simulink model "assignment5"  (R2017b)
settings: Solver=VariableStepAuto  StartTime=0.0  StopTime=10.0  RelTol=1e-3
libraries: hdlsllib x17
settings Model: Creator=Raymond  LastModifiedBy=Ray

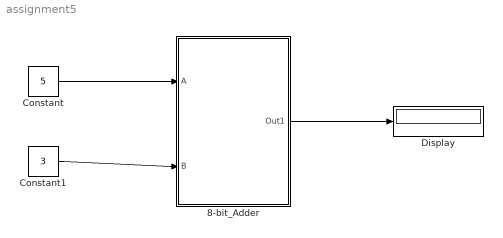
== system assignment5 ==
  8-bit_Adder : Subsystem
  Constant : Constant  Value=5  OutDataTypeStr=int8  SampleTime=-1
  Constant1 : Constant  Value=3  OutDataTypeStr=int8  SampleTime=-1
  Display : Display
  wires:
  Constant/1 -> 8-bit_Adder/1(A)
  Constant1/1 -> 8-bit_Adder/2(B)
  8-bit_Adder/1(Out1) -> Display/1

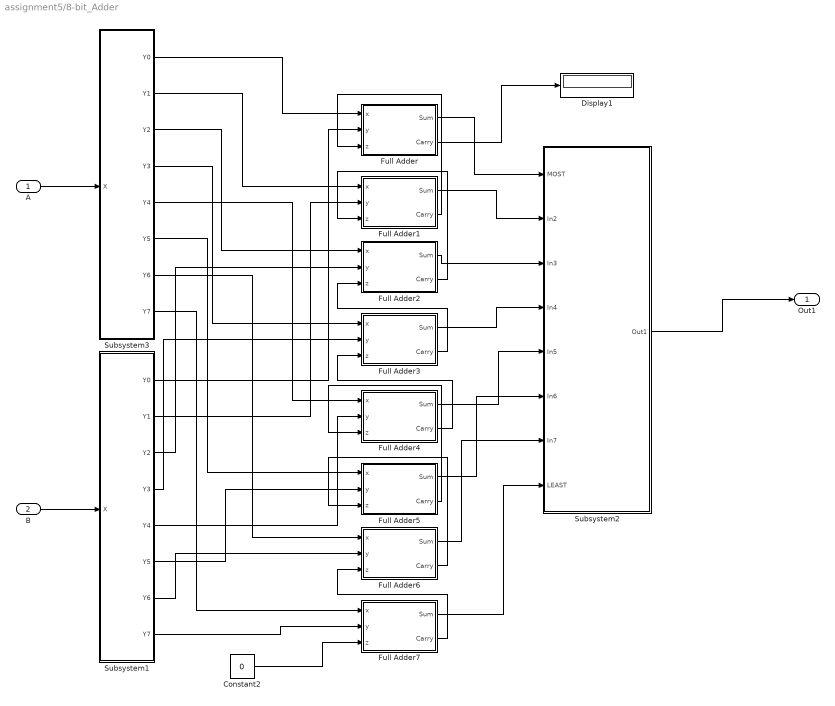
== system assignment5/8-bit_Adder ==
  A : Inport
  B : Inport  Port=2
  Constant2 : Constant  Value=0  OutDataTypeStr=int8  SampleTime=-1
  Display1 : Display
  Full Adder : Subsystem
  Full Adder1 : Subsystem
  Full Adder2 : Subsystem
  Full Adder3 : Subsystem
  Full Adder4 : Subsystem
  Full Adder5 : Subsystem
  Full Adder6 : Subsystem
  Full Adder7 : Subsystem
  Subsystem1 : Subsystem
  Subsystem2 : Subsystem
  Subsystem3 : Subsystem
  Out1 : Outport
  wires:
  A/1 -> Subsystem3/1(X)
  B/1 -> Subsystem1/1(X)
  Subsystem3/1(Y0) -> Full Adder/1(x)
  Subsystem3/2(Y1) -> Full Adder1/1(x)
  Subsystem3/3(Y2) -> Full Adder2/1(x)
  Subsystem3/4(Y3) -> Full Adder3/1(x)
  Subsystem3/5(Y4) -> Full Adder4/1(x)
  Subsystem3/6(Y5) -> Full Adder5/1(x)
  Subsystem3/7(Y6) -> Full Adder6/1(x)
  Subsystem3/8(Y7) -> Full Adder7/1(x)
  Subsystem1/1(Y0) -> Full Adder/2(y)
  Subsystem1/2(Y1) -> Full Adder1/2(y)
  Subsystem1/3(Y2) -> Full Adder2/2(y)
  Subsystem1/4(Y3) -> Full Adder3/2(y)
  Subsystem1/5(Y4) -> Full Adder4/2(y)
  Subsystem1/6(Y5) -> Full Adder5/2(y)
  Subsystem1/7(Y6) -> Full Adder6/2(y)
  Subsystem1/8(Y7) -> Full Adder7/2(y)
  Constant2/1 -> Full Adder7/3(z)
  Full Adder7/2(Carry) -> Full Adder6/3(z)
  Full Adder6/2(Carry) -> Full Adder5/3(z)
  Full Adder5/2(Carry) -> Full Adder4/3(z)
  Full Adder4/2(Carry) -> Full Adder3/3(z)
  Full Adder3/2(Carry) -> Full Adder2/3(z)
  Full Adder2/2(Carry) -> Full Adder1/3(z)
  Full Adder1/2(Carry) -> Full Adder/3(z)
  Subsystem2/1(Out1) -> Out1/1
  Full Adder/2(Carry) -> Display1/1
  Full Adder2/1(Sum) -> Subsystem2/3(In3)
  Full Adder3/1(Sum) -> Subsystem2/4(In4)
  Full Adder1/1(Sum) -> Subsystem2/2(In2)
  Full Adder4/1(Sum) -> Subsystem2/5(In5)
  Full Adder/1(Sum) -> Subsystem2/1(MOST)
  Full Adder5/1(Sum) -> Subsystem2/6(In6)
  Full Adder6/1(Sum) -> Subsystem2/7(In7)
  Full Adder7/1(Sum) -> Subsystem2/8(LEAST)

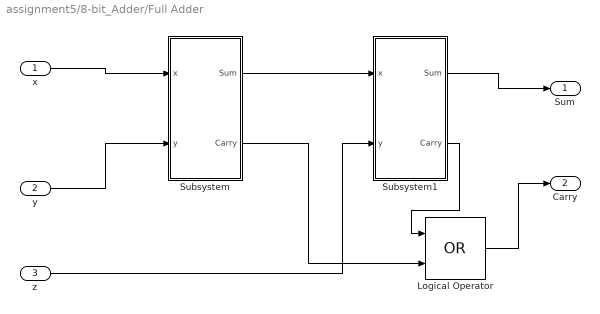
== system assignment5/8-bit_Adder/Full Adder ==
  x : Inport
  y : Inport  Port=2
  z : Inport  Port=3
  Logical Operator : Logic  Operator=OR  IconShape=distinctive  AllPortsSameDT=off  OutDataTypeStr=boolean
  Subsystem : Subsystem
  Subsystem1 : Subsystem
  Sum : Outport
  Carry : Outport  Port=2
  wires:
  z/1 -> Subsystem1/2(y)
  Subsystem/2(Carry) -> Logical Operator/2
  Subsystem1/1(Sum) -> Sum/1
  x/1 -> Subsystem/1(x)
  y/1 -> Subsystem/2(y)
  Subsystem/1(Sum) -> Subsystem1/1(x)
  Subsystem1/2(Carry) -> Logical Operator/1
  Logical Operator/1 -> Carry/1

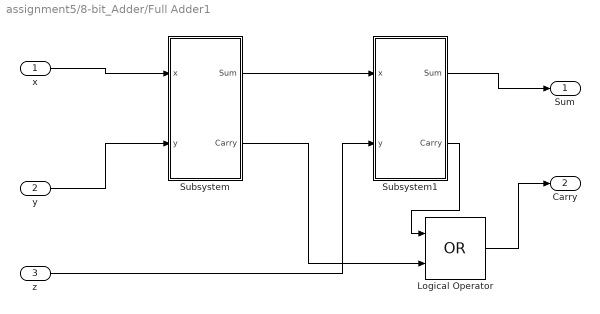
== system assignment5/8-bit_Adder/Full Adder1 ==
  x : Inport
  y : Inport  Port=2
  z : Inport  Port=3
  Logical Operator : Logic  Operator=OR  IconShape=distinctive  AllPortsSameDT=off  OutDataTypeStr=boolean
  Subsystem : Subsystem
  Subsystem1 : Subsystem
  Sum : Outport
  Carry : Outport  Port=2
  wires:
  z/1 -> Subsystem1/2(y)
  Subsystem/2(Carry) -> Logical Operator/2
  Subsystem1/1(Sum) -> Sum/1
  x/1 -> Subsystem/1(x)
  y/1 -> Subsystem/2(y)
  Subsystem/1(Sum) -> Subsystem1/1(x)
  Subsystem1/2(Carry) -> Logical Operator/1
  Logical Operator/1 -> Carry/1

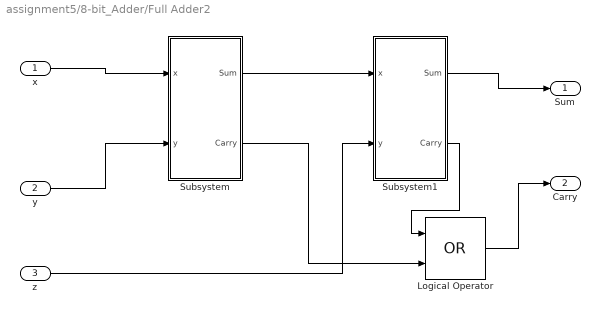
== system assignment5/8-bit_Adder/Full Adder2 ==
  x : Inport
  y : Inport  Port=2
  z : Inport  Port=3
  Logical Operator : Logic  Operator=OR  IconShape=distinctive  AllPortsSameDT=off  OutDataTypeStr=boolean
  Subsystem : Subsystem
  Subsystem1 : Subsystem
  Sum : Outport
  Carry : Outport  Port=2
  wires:
  z/1 -> Subsystem1/2(y)
  Subsystem/2(Carry) -> Logical Operator/2
  Subsystem1/1(Sum) -> Sum/1
  x/1 -> Subsystem/1(x)
  y/1 -> Subsystem/2(y)
  Subsystem/1(Sum) -> Subsystem1/1(x)
  Subsystem1/2(Carry) -> Logical Operator/1
  Logical Operator/1 -> Carry/1

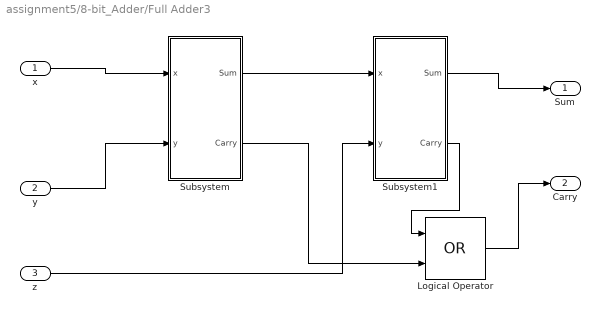
== system assignment5/8-bit_Adder/Full Adder3 ==
  x : Inport
  y : Inport  Port=2
  z : Inport  Port=3
  Logical Operator : Logic  Operator=OR  IconShape=distinctive  AllPortsSameDT=off  OutDataTypeStr=boolean
  Subsystem : Subsystem
  Subsystem1 : Subsystem
  Sum : Outport
  Carry : Outport  Port=2
  wires:
  Logical Operator/1 -> Carry/1
  Subsystem1/2(Carry) -> Logical Operator/1
  Subsystem/1(Sum) -> Subsystem1/1(x)
  y/1 -> Subsystem/2(y)
  x/1 -> Subsystem/1(x)
  Subsystem1/1(Sum) -> Sum/1
  Subsystem/2(Carry) -> Logical Operator/2
  z/1 -> Subsystem1/2(y)

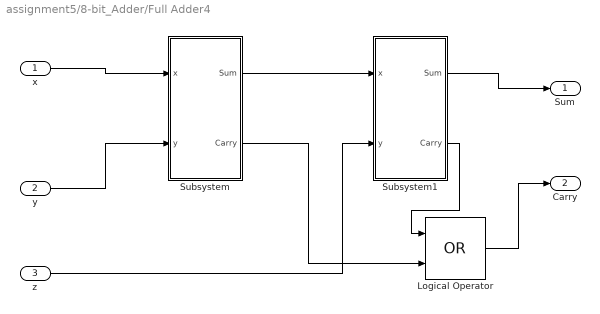
== system assignment5/8-bit_Adder/Full Adder4 ==
  x : Inport
  y : Inport  Port=2
  z : Inport  Port=3
  Logical Operator : Logic  Operator=OR  IconShape=distinctive  AllPortsSameDT=off  OutDataTypeStr=boolean
  Subsystem : Subsystem
  Subsystem1 : Subsystem
  Sum : Outport
  Carry : Outport  Port=2
  wires:
  z/1 -> Subsystem1/2(y)
  Subsystem/2(Carry) -> Logical Operator/2
  Subsystem1/1(Sum) -> Sum/1
  x/1 -> Subsystem/1(x)
  y/1 -> Subsystem/2(y)
  Subsystem/1(Sum) -> Subsystem1/1(x)
  Subsystem1/2(Carry) -> Logical Operator/1
  Logical Operator/1 -> Carry/1

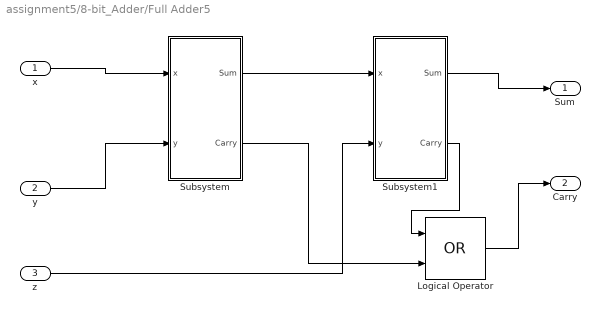
== system assignment5/8-bit_Adder/Full Adder5 ==
  x : Inport
  y : Inport  Port=2
  z : Inport  Port=3
  Logical Operator : Logic  Operator=OR  IconShape=distinctive  AllPortsSameDT=off  OutDataTypeStr=boolean
  Subsystem : Subsystem
  Subsystem1 : Subsystem
  Sum : Outport
  Carry : Outport  Port=2
  wires:
  z/1 -> Subsystem1/2(y)
  Subsystem/2(Carry) -> Logical Operator/2
  Subsystem1/1(Sum) -> Sum/1
  x/1 -> Subsystem/1(x)
  y/1 -> Subsystem/2(y)
  Subsystem/1(Sum) -> Subsystem1/1(x)
  Subsystem1/2(Carry) -> Logical Operator/1
  Logical Operator/1 -> Carry/1

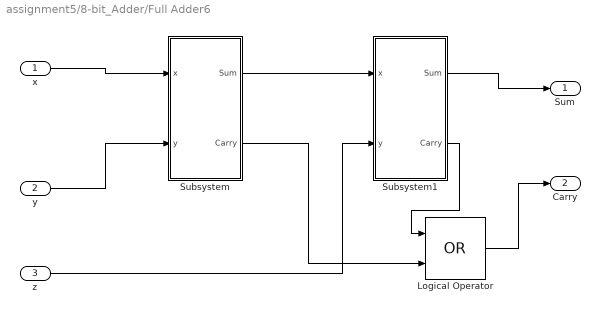
== system assignment5/8-bit_Adder/Full Adder6 ==
  x : Inport
  y : Inport  Port=2
  z : Inport  Port=3
  Logical Operator : Logic  Operator=OR  IconShape=distinctive  AllPortsSameDT=off  OutDataTypeStr=boolean
  Subsystem : Subsystem
  Subsystem1 : Subsystem
  Sum : Outport
  Carry : Outport  Port=2
  wires:
  z/1 -> Subsystem1/2(y)
  Subsystem/2(Carry) -> Logical Operator/2
  Subsystem1/1(Sum) -> Sum/1
  x/1 -> Subsystem/1(x)
  y/1 -> Subsystem/2(y)
  Subsystem/1(Sum) -> Subsystem1/1(x)
  Subsystem1/2(Carry) -> Logical Operator/1
  Logical Operator/1 -> Carry/1

== system assignment5/8-bit_Adder/Full Adder7 ==
  x : Inport
  y : Inport  Port=2
  z : Inport  Port=3
  Logical Operator : Logic  Operator=OR  IconShape=distinctive  AllPortsSameDT=off  OutDataTypeStr=boolean
  Subsystem : Subsystem
  Subsystem1 : Subsystem
  Sum : Outport
  Carry : Outport  Port=2
  wires:
  Logical Operator/1 -> Carry/1
  Subsystem1/2(Carry) -> Logical Operator/1
  Subsystem/1(Sum) -> Subsystem1/1(x)
  y/1 -> Subsystem/2(y)
  x/1 -> Subsystem/1(x)
  Subsystem1/1(Sum) -> Sum/1
  Subsystem/2(Carry) -> Logical Operator/2
  z/1 -> Subsystem1/2(y)

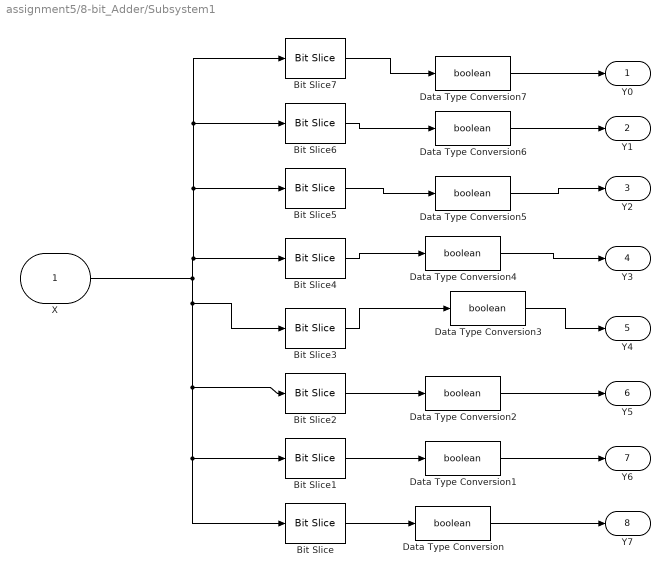
== system assignment5/8-bit_Adder/Subsystem1 ==
  X : Inport  OutDataTypeStr=int8  SampleTime=1
  Bit Slice : hdlsllib/Logic and Bit Operations/Bit Slice  lidx=0  ridx=0
  Bit Slice1 : hdlsllib/Logic and Bit Operations/Bit Slice  lidx=1  ridx=1
  Bit Slice2 : hdlsllib/Logic and Bit Operations/Bit Slice  lidx=2  ridx=2
  Bit Slice3 : hdlsllib/Logic and Bit Operations/Bit Slice  lidx=3  ridx=3
  Bit Slice4 : hdlsllib/Logic and Bit Operations/Bit Slice  lidx=4  ridx=4
  Bit Slice5 : hdlsllib/Logic and Bit Operations/Bit Slice  lidx=5  ridx=5
  Bit Slice6 : hdlsllib/Logic and Bit Operations/Bit Slice  lidx=6  ridx=6
  Bit Slice7 : hdlsllib/Logic and Bit Operations/Bit Slice  lidx=7  ridx=7
  Data Type Conversion{,1..7} (8 alike) : DataTypeConversion  OutDataTypeStr=boolean
  Y0 : Outport
  Y1 : Outport  Port=2
  Y2 : Outport  Port=3
  Y3 : Outport  Port=4
  Y4 : Outport  Port=5
  Y5 : Outport  Port=6
  Y6 : Outport  Port=7
  Y7 : Outport  Port=8
  wires:
  Data Type Conversion/1 -> Y7/1
  Data Type Conversion1/1 -> Y6/1
  Data Type Conversion6/1 -> Y1/1
  Bit Slice5/1 -> Data Type Conversion5/1
  Data Type Conversion5/1 -> Y2/1
  Data Type Conversion7/1 -> Y0/1
  X/1 -> Bit Slice/1, Bit Slice1/1, Bit Slice2/1, Bit Slice3/1, Bit Slice4/1, Bit Slice5/1, Bit Slice7/1, Bit Slice6/1
  Data Type Conversion3/1 -> Y4/1
  Data Type Conversion4/1 -> Y3/1
  Bit Slice2/1 -> Data Type Conversion2/1
  Bit Slice1/1 -> Data Type Conversion1/1
  Bit Slice/1 -> Data Type Conversion/1
  Data Type Conversion2/1 -> Y5/1
  Bit Slice7/1 -> Data Type Conversion7/1
  Bit Slice6/1 -> Data Type Conversion6/1
  Bit Slice4/1 -> Data Type Conversion4/1
  Bit Slice3/1 -> Data Type Conversion3/1

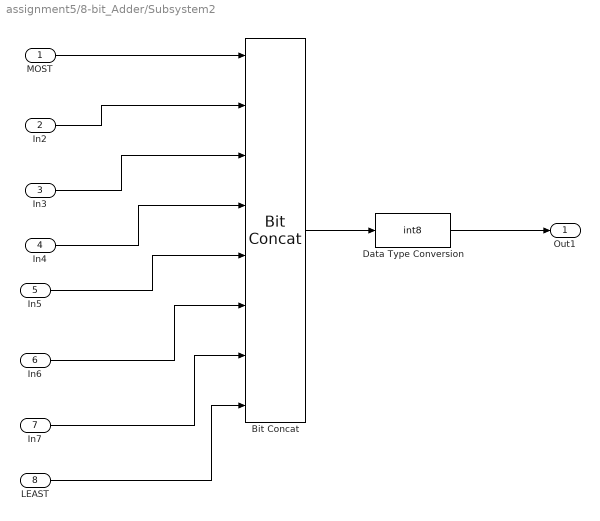
== system assignment5/8-bit_Adder/Subsystem2 ==
  MOST : Inport
  In2 : Inport  Port=2
  In3 : Inport  Port=3
  In4 : Inport  Port=4
  In5 : Inport  Port=5
  In6 : Inport  Port=6
  In7 : Inport  Port=7
  LEAST : Inport  Port=8
  Bit Concat : hdlsllib/Logic and Bit Operations/Bit Concat  numInputs=8
      settings: SourceProductName=HDL Coder  SourceProductBaseCode=HD
  Data Type Conversion : DataTypeConversion  OutDataTypeStr=int8
  Out1 : Outport
  wires:
  Bit Concat/1 -> Data Type Conversion/1
  Data Type Conversion/1 -> Out1/1
  In5/1 -> Bit Concat/5
  In6/1 -> Bit Concat/6
  MOST/1 -> Bit Concat/1
  In7/1 -> Bit Concat/7
  In3/1 -> Bit Concat/3
  In4/1 -> Bit Concat/4
  LEAST/1 -> Bit Concat/8
  In2/1 -> Bit Concat/2

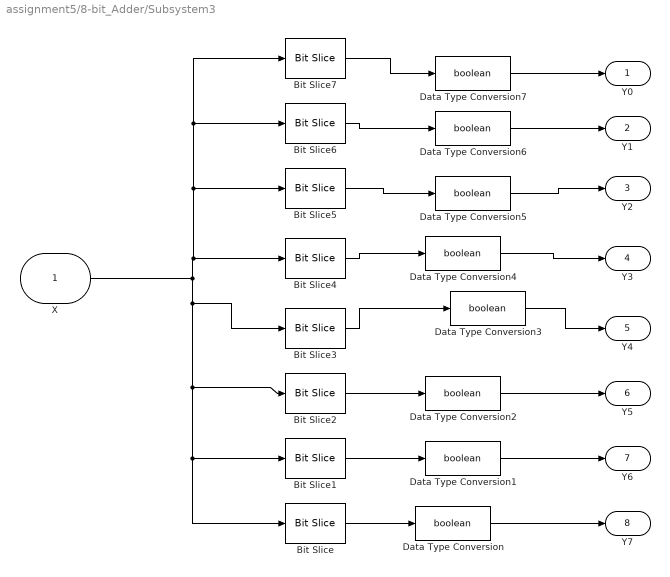
== system assignment5/8-bit_Adder/Subsystem3 ==
  X : Inport  OutDataTypeStr=int8  SampleTime=1
  Bit Slice : hdlsllib/Logic and Bit Operations/Bit Slice  lidx=0  ridx=0
  Bit Slice1 : hdlsllib/Logic and Bit Operations/Bit Slice  lidx=1  ridx=1
  Bit Slice2 : hdlsllib/Logic and Bit Operations/Bit Slice  lidx=2  ridx=2
  Bit Slice3 : hdlsllib/Logic and Bit Operations/Bit Slice  lidx=3  ridx=3
  Bit Slice4 : hdlsllib/Logic and Bit Operations/Bit Slice  lidx=4  ridx=4
  Bit Slice5 : hdlsllib/Logic and Bit Operations/Bit Slice  lidx=5  ridx=5
  Bit Slice6 : hdlsllib/Logic and Bit Operations/Bit Slice  lidx=6  ridx=6
  Bit Slice7 : hdlsllib/Logic and Bit Operations/Bit Slice  lidx=7  ridx=7
  Data Type Conversion{,1..7} (8 alike) : DataTypeConversion  OutDataTypeStr=boolean
  Y0 : Outport
  Y1 : Outport  Port=2
  Y2 : Outport  Port=3
  Y3 : Outport  Port=4
  Y4 : Outport  Port=5
  Y5 : Outport  Port=6
  Y6 : Outport  Port=7
  Y7 : Outport  Port=8
  wires:
  Data Type Conversion/1 -> Y7/1
  Data Type Conversion1/1 -> Y6/1
  Data Type Conversion6/1 -> Y1/1
  Bit Slice5/1 -> Data Type Conversion5/1
  Data Type Conversion5/1 -> Y2/1
  Data Type Conversion7/1 -> Y0/1
  X/1 -> Bit Slice/1, Bit Slice1/1, Bit Slice2/1, Bit Slice3/1, Bit Slice4/1, Bit Slice5/1, Bit Slice7/1, Bit Slice6/1
  Data Type Conversion3/1 -> Y4/1
  Data Type Conversion4/1 -> Y3/1
  Bit Slice2/1 -> Data Type Conversion2/1
  Bit Slice1/1 -> Data Type Conversion1/1
  Bit Slice/1 -> Data Type Conversion/1
  Data Type Conversion2/1 -> Y5/1
  Bit Slice7/1 -> Data Type Conversion7/1
  Bit Slice6/1 -> Data Type Conversion6/1
  Bit Slice4/1 -> Data Type Conversion4/1
  Bit Slice3/1 -> Data Type Conversion3/1

== system assignment5/8-bit_Adder/Full Adder/Subsystem ==
  x : Inport
  y : Inport  Port=2
  Logical Operator : Logic  IconShape=distinctive  AllPortsSameDT=off  OutDataTypeStr=boolean
  Logical Operator1 : Logic  Operator=XOR  IconShape=distinctive  AllPortsSameDT=off  OutDataTypeStr=boolean
  Sum : Outport
  Carry : Outport  Port=2
  wires:
  x/1 -> Logical Operator/1, Logical Operator1/1
  y/1 -> Logical Operator1/2, Logical Operator/2
  Logical Operator/1 -> Carry/1
  Logical Operator1/1 -> Sum/1

== system assignment5/8-bit_Adder/Full Adder/Subsystem1 ==
  x : Inport
  y : Inport  Port=2
  Logical Operator : Logic  IconShape=distinctive  AllPortsSameDT=off  OutDataTypeStr=boolean
  Logical Operator1 : Logic  Operator=XOR  IconShape=distinctive  AllPortsSameDT=off  OutDataTypeStr=boolean
  Sum : Outport
  Carry : Outport  Port=2
  wires:
  x/1 -> Logical Operator/1, Logical Operator1/1
  y/1 -> Logical Operator1/2, Logical Operator/2
  Logical Operator/1 -> Carry/1
  Logical Operator1/1 -> Sum/1

== system assignment5/8-bit_Adder/Full Adder1/Subsystem ==
  x : Inport
  y : Inport  Port=2
  Logical Operator : Logic  IconShape=distinctive  AllPortsSameDT=off  OutDataTypeStr=boolean
  Logical Operator1 : Logic  Operator=XOR  IconShape=distinctive  AllPortsSameDT=off  OutDataTypeStr=boolean
  Sum : Outport
  Carry : Outport  Port=2
  wires:
  x/1 -> Logical Operator/1, Logical Operator1/1
  y/1 -> Logical Operator1/2, Logical Operator/2
  Logical Operator/1 -> Carry/1
  Logical Operator1/1 -> Sum/1

== system assignment5/8-bit_Adder/Full Adder1/Subsystem1 ==
  x : Inport
  y : Inport  Port=2
  Logical Operator : Logic  IconShape=distinctive  AllPortsSameDT=off  OutDataTypeStr=boolean
  Logical Operator1 : Logic  Operator=XOR  IconShape=distinctive  AllPortsSameDT=off  OutDataTypeStr=boolean
  Sum : Outport
  Carry : Outport  Port=2
  wires:
  x/1 -> Logical Operator/1, Logical Operator1/1
  y/1 -> Logical Operator1/2, Logical Operator/2
  Logical Operator/1 -> Carry/1
  Logical Operator1/1 -> Sum/1

== system assignment5/8-bit_Adder/Full Adder2/Subsystem ==
  x : Inport
  y : Inport  Port=2
  Logical Operator : Logic  IconShape=distinctive  AllPortsSameDT=off  OutDataTypeStr=boolean
  Logical Operator1 : Logic  Operator=XOR  IconShape=distinctive  AllPortsSameDT=off  OutDataTypeStr=boolean
  Sum : Outport
  Carry : Outport  Port=2
  wires:
  x/1 -> Logical Operator/1, Logical Operator1/1
  y/1 -> Logical Operator1/2, Logical Operator/2
  Logical Operator/1 -> Carry/1
  Logical Operator1/1 -> Sum/1

== system assignment5/8-bit_Adder/Full Adder2/Subsystem1 ==
  x : Inport
  y : Inport  Port=2
  Logical Operator : Logic  IconShape=distinctive  AllPortsSameDT=off  OutDataTypeStr=boolean
  Logical Operator1 : Logic  Operator=XOR  IconShape=distinctive  AllPortsSameDT=off  OutDataTypeStr=boolean
  Sum : Outport
  Carry : Outport  Port=2
  wires:
  x/1 -> Logical Operator/1, Logical Operator1/1
  y/1 -> Logical Operator1/2, Logical Operator/2
  Logical Operator/1 -> Carry/1
  Logical Operator1/1 -> Sum/1

== system assignment5/8-bit_Adder/Full Adder3/Subsystem ==
  x : Inport
  y : Inport  Port=2
  Logical Operator : Logic  IconShape=distinctive  AllPortsSameDT=off  OutDataTypeStr=boolean
  Logical Operator1 : Logic  Operator=XOR  IconShape=distinctive  AllPortsSameDT=off  OutDataTypeStr=boolean
  Sum : Outport
  Carry : Outport  Port=2
  wires:
  Logical Operator1/1 -> Sum/1
  Logical Operator/1 -> Carry/1
  y/1 -> Logical Operator/2, Logical Operator1/2
  x/1 -> Logical Operator1/1, Logical Operator/1

== system assignment5/8-bit_Adder/Full Adder3/Subsystem1 ==
  x : Inport
  y : Inport  Port=2
  Logical Operator : Logic  IconShape=distinctive  AllPortsSameDT=off  OutDataTypeStr=boolean
  Logical Operator1 : Logic  Operator=XOR  IconShape=distinctive  AllPortsSameDT=off  OutDataTypeStr=boolean
  Sum : Outport
  Carry : Outport  Port=2
  wires:
  Logical Operator1/1 -> Sum/1
  Logical Operator/1 -> Carry/1
  y/1 -> Logical Operator/2, Logical Operator1/2
  x/1 -> Logical Operator1/1, Logical Operator/1

== system assignment5/8-bit_Adder/Full Adder4/Subsystem ==
  x : Inport
  y : Inport  Port=2
  Logical Operator : Logic  IconShape=distinctive  AllPortsSameDT=off  OutDataTypeStr=boolean
  Logical Operator1 : Logic  Operator=XOR  IconShape=distinctive  AllPortsSameDT=off  OutDataTypeStr=boolean
  Sum : Outport
  Carry : Outport  Port=2
  wires:
  x/1 -> Logical Operator/1, Logical Operator1/1
  y/1 -> Logical Operator1/2, Logical Operator/2
  Logical Operator/1 -> Carry/1
  Logical Operator1/1 -> Sum/1

== system assignment5/8-bit_Adder/Full Adder4/Subsystem1 ==
  x : Inport
  y : Inport  Port=2
  Logical Operator : Logic  IconShape=distinctive  AllPortsSameDT=off  OutDataTypeStr=boolean
  Logical Operator1 : Logic  Operator=XOR  IconShape=distinctive  AllPortsSameDT=off  OutDataTypeStr=boolean
  Sum : Outport
  Carry : Outport  Port=2
  wires:
  x/1 -> Logical Operator/1, Logical Operator1/1
  y/1 -> Logical Operator1/2, Logical Operator/2
  Logical Operator/1 -> Carry/1
  Logical Operator1/1 -> Sum/1

== system assignment5/8-bit_Adder/Full Adder5/Subsystem ==
  x : Inport
  y : Inport  Port=2
  Logical Operator : Logic  IconShape=distinctive  AllPortsSameDT=off  OutDataTypeStr=boolean
  Logical Operator1 : Logic  Operator=XOR  IconShape=distinctive  AllPortsSameDT=off  OutDataTypeStr=boolean
  Sum : Outport
  Carry : Outport  Port=2
  wires:
  x/1 -> Logical Operator/1, Logical Operator1/1
  y/1 -> Logical Operator1/2, Logical Operator/2
  Logical Operator/1 -> Carry/1
  Logical Operator1/1 -> Sum/1

== system assignment5/8-bit_Adder/Full Adder5/Subsystem1 ==
  x : Inport
  y : Inport  Port=2
  Logical Operator : Logic  IconShape=distinctive  AllPortsSameDT=off  OutDataTypeStr=boolean
  Logical Operator1 : Logic  Operator=XOR  IconShape=distinctive  AllPortsSameDT=off  OutDataTypeStr=boolean
  Sum : Outport
  Carry : Outport  Port=2
  wires:
  x/1 -> Logical Operator/1, Logical Operator1/1
  y/1 -> Logical Operator1/2, Logical Operator/2
  Logical Operator/1 -> Carry/1
  Logical Operator1/1 -> Sum/1

== system assignment5/8-bit_Adder/Full Adder6/Subsystem ==
  x : Inport
  y : Inport  Port=2
  Logical Operator : Logic  IconShape=distinctive  AllPortsSameDT=off  OutDataTypeStr=boolean
  Logical Operator1 : Logic  Operator=XOR  IconShape=distinctive  AllPortsSameDT=off  OutDataTypeStr=boolean
  Sum : Outport
  Carry : Outport  Port=2
  wires:
  x/1 -> Logical Operator/1, Logical Operator1/1
  y/1 -> Logical Operator1/2, Logical Operator/2
  Logical Operator/1 -> Carry/1
  Logical Operator1/1 -> Sum/1

== system assignment5/8-bit_Adder/Full Adder6/Subsystem1 ==
  x : Inport
  y : Inport  Port=2
  Logical Operator : Logic  IconShape=distinctive  AllPortsSameDT=off  OutDataTypeStr=boolean
  Logical Operator1 : Logic  Operator=XOR  IconShape=distinctive  AllPortsSameDT=off  OutDataTypeStr=boolean
  Sum : Outport
  Carry : Outport  Port=2
  wires:
  x/1 -> Logical Operator/1, Logical Operator1/1
  y/1 -> Logical Operator1/2, Logical Operator/2
  Logical Operator/1 -> Carry/1
  Logical Operator1/1 -> Sum/1

== system assignment5/8-bit_Adder/Full Adder7/Subsystem ==
  x : Inport
  y : Inport  Port=2
  Logical Operator : Logic  IconShape=distinctive  AllPortsSameDT=off  OutDataTypeStr=boolean
  Logical Operator1 : Logic  Operator=XOR  IconShape=distinctive  AllPortsSameDT=off  OutDataTypeStr=boolean
  Sum : Outport
  Carry : Outport  Port=2
  wires:
  Logical Operator1/1 -> Sum/1
  Logical Operator/1 -> Carry/1
  y/1 -> Logical Operator/2, Logical Operator1/2
  x/1 -> Logical Operator1/1, Logical Operator/1

== system assignment5/8-bit_Adder/Full Adder7/Subsystem1 ==
  x : Inport
  y : Inport  Port=2
  Logical Operator : Logic  IconShape=distinctive  AllPortsSameDT=off  OutDataTypeStr=boolean
  Logical Operator1 : Logic  Operator=XOR  IconShape=distinctive  AllPortsSameDT=off  OutDataTypeStr=boolean
  Sum : Outport
  Carry : Outport  Port=2
  wires:
  Logical Operator1/1 -> Sum/1
  Logical Operator/1 -> Carry/1
  y/1 -> Logical Operator/2, Logical Operator1/2
  x/1 -> Logical Operator1/1, Logical Operator/1
